simulink model "DBMPCC"  (R2022a)
settings: Solver=ode1  StartTime=0.0  StopTime=Inf  FixedStep=Ts  RelTol=1e-3  EnableMultiTasking=on
PostLoadFcn:
  | , if any(exist('dsrtsu_mdlpostloadfcn', 'file') ~= 0), dsrtsu_mdlpostloadfcn('Execute', bdroot); end,
InitFcn:
  | , if any(exist('rtifpga_mdlclblib', 'file') ~= 0), rtifpga_mdlclblib('Init', bdroot); end,
undefined symbols (not defined in the file): Ls, P, Ts
libraries: rtilib1104 x15, rtitasklib x1
settings Model: DSRTSU_INTERNAL_RTI_VER=600  DSRTSU_INTERNAL_RTI_TYPE=rti1104  DSRTSU_INTERNAL_RTIFPGA=180  DSRTSU_INTERNAL_RTISTBM_VER=1.4.4  SimulationMode=external  Creator=Admin  LastModifiedBy=acer
settings SolverCC: AlgebraicLoopSolver=TrustRegion
settings DataIOCC: LimitDataPoints=on  SaveFormat=Array  SignalLoggingSaveFormat=ModelDataLogs  ReturnWorkspaceOutputs=off
settings OptimizationCC: BlockReduction=off  OptimizeBlockIOStorage=off  BufferReuse=off  GlobalBufferReuse=off  ExpressionFolding=off  ExpressionDepthLimit=2147483647  LocalBlockOutputs=off  LifeSpan=inf
settings DebuggingCC: UnderspecifiedInitializationDetection=Classic  MergeDetectMultiDrivingBlocksExec=none  SolverPrmCheckMsg=warning  FcnCallInpInsideContextMsg=warning  UnconnectedInputMsg=warning  UnconnectedOutputMsg=warning  UnconnectedLineMsg=warning  StateNameClashWarn=warning  SFUnexpectedBacktrackingDiag=warning  SFNoUnconditionalDefaultTransitionDiag=warning  SFExecutionAtInitializationDiag=none  SFMachineParentedDataDiag=warning  ArithmeticOperatorsInVariantConditions=warning
settings HardwareCC: ProdBitPerPointer=32  ProdBitPerSizeT=32  ProdBitPerPtrDiffT=32  ProdLargestAtomicInteger=Integer  ProdEndianess=BigEndian  ProdWordSize=32  ProdHWDeviceType=Custom Processor->Custom  TargetIntDivRoundTo=Zero  TargetEndianess=BigEndian  TargetHWDeviceType=Custom Processor->Custom
settings ModelReferenceCC: PropagateSignalLabelsOutOfModel=off
settings SFSimCC: SimUseLocalCustomCode=off  MATLABDynamicMemAlloc=off  CustomCodeUndefinedFunction=UseInterfaceOnly
settings RTWCC: Description=dSPACE DS1104 Hardware Platform  SystemTargetFile=rti1104.tlc  MakeCommand=make_rti  TemplateMakefile=rti1104.tmf  RTWUseLocalCustomCode=off
settings CodeAppCC: StateflowObjectComments=on
settings STFCustomTargetCC: ParMdlRefBuildCompliant=on  GRTInterface=off  SystemTargetFile=rti1104.tlc
settings GRTTargetCC: TargetLangStandard=C89/C90 (ANSI)  CompOptLevelCompliant=off  ConcurrentExecutionCompliant=off  CombineOutputUpdateFcns=off  MatFileLogging=off  CPPClassGenCompliant=off  UseToolchainInfoCompliant=off  ExtModeMexFile=noextcomm
settings ConfigComp: CovMetricSettings=dw  CovSaveCumulativeToWorkspaceVar=on  CovSaveSingleToWorkspaceVar=on  CovExternalEMLEnable=off

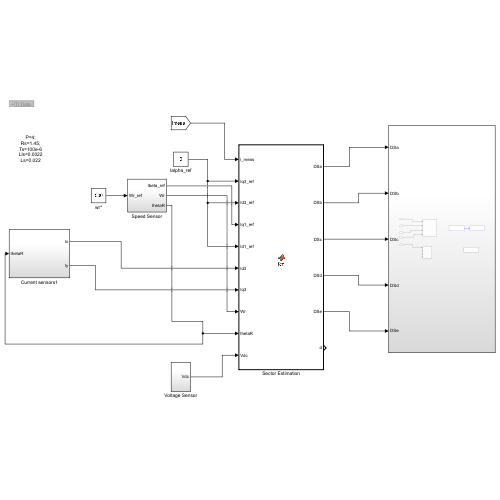
[thumbnail: Simulink's stored preview of the top-level diagram]
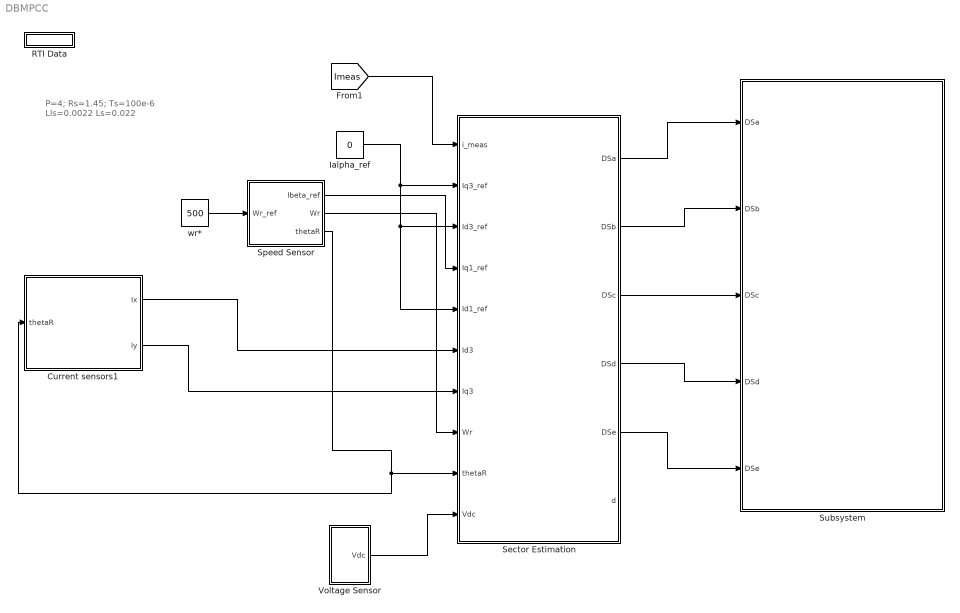
== system DBMPCC ==
  note: P=4;
      | Rs=1.45;
      | Ts=100e-6
      | Lls=0.0022
      | Ls=0.022
  Current sensors1 : Subsystem
  Ialpha_ref : Constant  Value=0
  RTI Data : Subsystem  Tag=struct('RTIDataServer',struct('RTIDataServerVs','2','RTIModelDescription','struct(''main'',''FP_CONV_PCC_SF_30V_PWM_n_duty_CurrErr'',''sub'','''',''isMp'',0)'))  LoadFcn="if exist('rtidc'), try,  rtidc('DataHostBlockClbLoad', gcbh); catch, disp(['Warning: ''LoadFcn'' for RTI Data block failed: ' lasterr]); end, end,"  mask(RTI_DATA_HOST){}
      mask help:
      | RTI Data Block.
      | This block is used by RTI to store internal model-dependent data.
      | Please keep this block on the root level of the model. Deleting this block will result in data loss.
      |
      | NEVER DELETE OR COPY THIS BLOCK!
      settings: CopyFcn="if exist('rtidc'), try,  rtidc('DataHostBlockClbCopy', gcbh); catch, disp(['Warning: ''CopyFcn'' for RTI Data block failed: ' lasterr]); end, end,"  DeleteFcn="if exist('rtidc'), try,  rtidc('DataHostBlockClbDelete', gcbh); catch, disp(['Warning: ''DeleteFcn'' for RTI Data block failed: ' lasterr]); end, end,"  ModelCloseFcn="if exist('rtidc'), try,  rtidc('DataHostBlockClbModelClose', gcbh); catch, disp(['Warning: ''ModelCloseFcn'' for RTI Data block failed: ' lasterr]); end, end,"  PreSaveFcn="if exist('rtidc'), try,  rtidc('DataHostBlockClbPreSave', gcbh); catch, disp(['Warning: ''PreSaveFcn'' for RTI Data block failed: ' lasterr]); end, end,"  PostSaveFcn="if exist('rtidc'), try,  rtidc('DataHostBlockClbPostSave', gcbh); catch, disp(['Warning: ''PostSaveFcn'' for RTI Data block failed: ' lasterr]); end, end,"  NameChangeFcn="if exist('rtidc'), try,  rtidc('DataHostBlockClbNameChange', gcbh); catch, disp(['Warning: ''NameChangeFcn'' for RTI Data block failed: ' lasterr]); end, end,"
      mask Help:
      | RTI Data Block.
      | This block is used by RTI to store internal model-dependent data.
      | Please keep this block on the root level of the model. Deleting this block will result in data loss.
      | 
      | NEVER DELETE OR COPY THIS BLOCK!
      mask Display:
      | text(0.5, 0.5, 'RTI Data', 'HorizontalAlignment', 'center');
      | plot([1 0]);
  Sector Estimation : MATLAB Function  TreatAsAtomicUnit=on  SystemSampleTime=Ts
  Speed Sensor : Subsystem
  Subsystem : Subsystem
  Voltage Sensor : Subsystem
  wr* : Constant  Value=500
  wires:
  Voltage Sensor/1(Vdc) -> Sector Estimation/10(Vdc)
  Ialpha_ref/1 -> Sector Estimation/2(Iq3_ref), Sector Estimation/3(Id3_ref), Sector Estimation/5(Id1_ref)
  wr*/1 -> Speed Sensor/1(Wr_ref)
  Speed Sensor/3(thetaR) -> Current sensors1/1(thetaR), Sector Estimation/9(thetaR)
  Speed Sensor/2(Wr) -> Sector Estimation/8(Wr)
  Speed Sensor/1(Ibeta_ref) -> Sector Estimation/4(Iq1_ref)
  [Imeas] -> Sector Estimation/1(i_meas)
  Current sensors1/1(Ix) -> Sector Estimation/6(Id3)
  Current sensors1/2(Iy) -> Sector Estimation/7(Iq3)
  Sector Estimation/1(DSa) -> Subsystem/1(DSa)
  Sector Estimation/2(DSb) -> Subsystem/2(DSb)
  Sector Estimation/3(DSc) -> Subsystem/3(DSc)
  Sector Estimation/4(DSd) -> Subsystem/4(DSd)
  Sector Estimation/5(DSe) -> Subsystem/5(DSe)

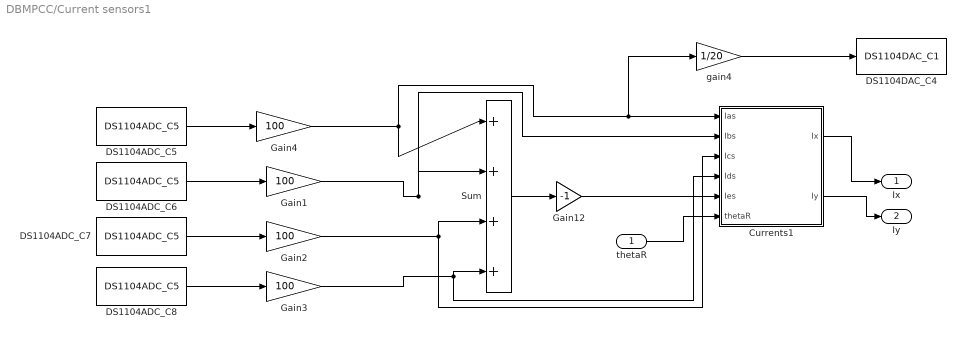
== system DBMPCC/Current sensors1 ==
  thetaR : Inport
  Currents1 : Subsystem
  DS1104ADC_C5 : rtilib1104/DS1104 MASTER PPC/DS1104ADC_C5  ChannelNo=5  TriggerMode=0  Reserved1=[]  Reserved2=[]  Reserved3=[]  Reserved4=[]  DialogFcn=gui1104adc  UnitName={ 'DS1104ADC_C' }  UnitValues={ 5 }  DSProperties=struct('RTI',struct('Version',uint32(1),'BlockType',struct('isSLSource',uint8(1),'isSLSink',uint8(0),'isHWSource',uint8(1),'isHWSink',uint8(0),'isSetup',uint8(0),'isInline',uint8(1),'isNonInline',uint8(0),'isInterrupt',uint8(0),'isChannelwise',uint8(1)),'IOBoardType','DS1104MASTER','UnitType','ADC','Identifier','ADC','DialogType','ML','BlockSet','NONE','SlaveProcessor','NONE'))
      settings: SourceProductName=dSPACE RTI1104
  DS1104ADC_C6 : rtilib1104/DS1104 MASTER PPC/DS1104ADC_C5  ChannelNo=6  TriggerMode=0  Reserved1=[]  Reserved2=[]  Reserved3=[]  Reserved4=[]  DialogFcn=gui1104adc  UnitName={ 'DS1104ADC_C' }  UnitValues={ 6 }  DSProperties=struct('RTI',struct('Version',uint32(1),'BlockType',struct('isSLSource',uint8(1),'isSLSink',uint8(0),'isHWSource',uint8(1),'isHWSink',uint8(0),'isSetup',uint8(0),'isInline',uint8(1),'isNonInline',uint8(0),'isInterrupt',uint8(0),'isChannelwise',uint8(1)),'IOBoardType','DS1104MASTER','UnitType','ADC','Identifier','ADC','DialogType','ML','BlockSet','NONE','SlaveProcessor','NONE'))
      settings: SourceProductName=dSPACE RTI1104
  DS1104ADC_C7 : rtilib1104/DS1104 MASTER PPC/DS1104ADC_C5  ChannelNo=7  TriggerMode=0  Reserved1=[]  Reserved2=[]  Reserved3=[]  Reserved4=[]  DialogFcn=gui1104adc  UnitName={ 'DS1104ADC_C' }  UnitValues={ 7 }  DSProperties=struct('RTI',struct('Version',uint32(1),'BlockType',struct('isSLSource',uint8(1),'isSLSink',uint8(0),'isHWSource',uint8(1),'isHWSink',uint8(0),'isSetup',uint8(0),'isInline',uint8(1),'isNonInline',uint8(0),'isInterrupt',uint8(0),'isChannelwise',uint8(1)),'IOBoardType','DS1104MASTER','UnitType','ADC','Identifier','ADC','DialogType','ML','BlockSet','NONE','SlaveProcessor','NONE'))
      settings: SourceProductName=dSPACE RTI1104
  DS1104ADC_C8 : rtilib1104/DS1104 MASTER PPC/DS1104ADC_C5  ChannelNo=8  TriggerMode=0  Reserved1=[]  Reserved2=[]  Reserved3=[]  Reserved4=[]  DialogFcn=gui1104adc  UnitName={ 'DS1104ADC_C' }  UnitValues={ 8 }  DSProperties=struct('RTI',struct('Version',uint32(1),'BlockType',struct('isSLSource',uint8(1),'isSLSink',uint8(0),'isHWSource',uint8(1),'isHWSink',uint8(0),'isSetup',uint8(0),'isInline',uint8(1),'isNonInline',uint8(0),'isInterrupt',uint8(0),'isChannelwise',uint8(1)),'IOBoardType','DS1104MASTER','UnitType','ADC','Identifier','ADC','DialogType','ML','BlockSet','NONE','SlaveProcessor','NONE'))
      settings: SourceProductName=dSPACE RTI1104
  DS1104DAC_C4 : rtilib1104/DS1104 MASTER PPC/DS1104DAC_C1  ChannelNo=4  InitValue=0  TermMode=0  TermValue=0  Reserved1=[]  Reserved2=[]  Reserved3=[]  Reserved4=[]  DialogFcn=gui1104dac  UnitName={ 'DS1104DAC_C'}  UnitValues={4}  DSProperties=struct('RTI',struct('Version',uint32(1),'BlockType',struct('isSLSource',uint8(0),'isSLSink',uint8(1),'isHWSource',uint8(0),'isHWSink',uint8(1),'isSetup',uint8(0),'isInline',uint8(1),'isNonInline',uint8(0),'isInterrupt',uint8(0),'isChannelwise',uint8(1)),'IOBoardType','DS1104MASTER','UnitType','DAC','Identifier','DAC','DialogType','ML','BlockSet','NONE','SlaveProcessor','NONE'))
      settings: SourceProductName=dSPACE RTI1104
  Gain{1..4} (4 alike) : Gain  Gain=100
  Gain12 : Gain  Gain=-1
  Sum : Sum  Inputs=|++++
  gain4 : Gain  Gain=1/20  SaturateOnIntegerOverflow=on  OutDataTypeStr=Inherit: Same as input  ParamDataTypeStr=Inherit: Same as input
  Ix : Outport
  Iy : Outport  Port=2
  wires:
  DS1104ADC_C5/1 -> Gain4/1
  DS1104ADC_C6/1 -> Gain1/1
  DS1104ADC_C7/1 -> Gain2/1
  DS1104ADC_C8/1 -> Gain3/1
  Sum/1 -> Gain12/1
  Gain12/1 -> Currents1/5(Ies)
  thetaR/1 -> Currents1/6(thetaR)
  Currents1/1(Ix) -> Ix/1
  Currents1/2(Iy) -> Iy/1
  Gain4/1 -> Sum/1, gain4/1, Currents1/1(Ias)
  Gain1/1 -> Currents1/2(Ibs), Sum/2
  Gain2/1 -> Currents1/3(Ics), Sum/3
  Gain3/1 -> Currents1/4(Ids), Sum/4
  gain4/1 -> DS1104DAC_C4/1

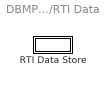
== system DBMPCC/RTI Data ==
  RTI Data Store : Subsystem  Tag="struct('private',struct('version',struct('dsVer',uint32(2),'dsVerCreation',uint32(2),'RTI',struct('ver','7.18','type','RTI1104')),'access',struct('type','Model','isPerm',1,'created',['03-Feb-2024 13:29:53'],'modified',['22-Jun-2024 12:50:59'],'location','')),'public',struct('main',struct('data',[]),'sub',struct('name',{{'FP_CONV_PCC_SF_30V_PWM_n_duty_CurrErr'}},'data',{{struct('TH',struct('thTaskInfo',struct('taskType',{'TIMER','HWINT','TMRINT','SWINT','GLINT'},'tasksNumOf',{1,0,0,0,0},'srcIds',{{'PWMINT'},{},{},{},{}},'taskNames',{{['Timer Task 1']},{},{},{},{}})),'th_tc',struct('dataType','TASK','taskGroupId','','taskGroupList',{{}},'taskSchedulingPolicy','FCFS','taskType','TIMER','blkh','FP_CONV_PCC_SF_30V_PWM_n_duty_CurrErr/Subsystem/DS1104SLAVE_PWMINT1','srcId','PWMINT','srcSgnName',['SLAVE-PWM-Interrupt with variable alignment'],'srcCpuName','','taskName',['Timer Task 1  [0.0001] s'],'taskNameDisplayExt','','smplTime',0.0001,'smplTimeOffs',0,'hasFixedPriority',0,'priority',1,'hasFixedOvc',0,'ovcType',1,'ovcMax',1),'tc_th',struct('dataType','TASK','taskGroupId','','taskGroupList',{{}},'taskSchedulingPolicy','FCFS','taskType','TIMER','blkh','FP_CONV_PCC_SF_30V_PWM_n_duty_CurrErr/Subsystem/DS1104SLAVE_PWMINT1','srcId','PWMINT','srcSgnName',['SLAVE-PWM-Interrupt with variable alignment'],'srcCpuName','','taskName',['Timer Task 1  [0.0001] s'],'taskNameDisplayExt','','smplTime',0.0001,'smplTimeOffs',0,'hasFixedPriority',0,'priority',1,'hasFixedOvc',0,'ovcType',1,'ovcMax',1))}})))"  mask(RTI_DATA_STORE){}
      mask help:
      | RTI Data Store Block. This block is used by RTI to store internal model dependent data. Deleting this block will result in data loss.
      |
      | NEVER DELETE, COPY, OR MODIFY THIS BLOCK!
      mask Help:
      | RTI Data Store Block. This block is used by RTI to store internal model dependent data. Deleting this block will result in data loss.
      | 
      | NEVER DELETE, COPY, OR MODIFY THIS BLOCK!
      mask Display: text(0.5, 0.5, ' ', 'HorizontalAlignment', 'center');

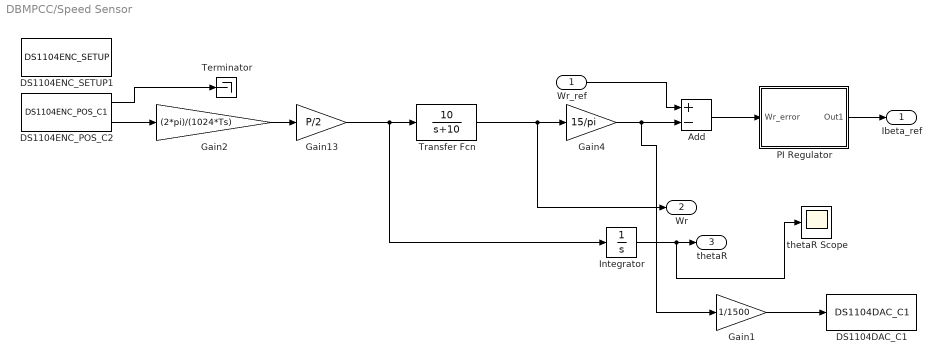
== system DBMPCC/Speed Sensor ==
  Wr_ref : Inport
  Add : Sum  Inputs=+-
  DS1104DAC_C1 : rtilib1104/DS1104 MASTER PPC/DS1104DAC_C1  ChannelNo=1  InitValue=0  TermMode=0  TermValue=0  Reserved1=[]  Reserved2=[]  Reserved3=[]  Reserved4=[]  DialogFcn=gui1104dac  UnitName={ 'DS1104DAC_C'}  UnitValues={ 1 }  DSProperties=struct('RTI',struct('Version',uint32(1),'BlockType',struct('isSLSource',uint8(0),'isSLSink',uint8(1),'isHWSource',uint8(0),'isHWSink',uint8(1),'isSetup',uint8(0),'isInline',uint8(1),'isNonInline',uint8(0),'isInterrupt',uint8(0),'isChannelwise',uint8(1)),'IOBoardType','DS1104MASTER','UnitType','DAC','Identifier','DAC','DialogType','ML','BlockSet','NONE','SlaveProcessor','NONE'))
      settings: SourceProductName=dSPACE RTI1104
  DS1104ENC_POS_C2 : rtilib1104/DS1104 MASTER PPC/DS1104ENC_POS_C1  ChannelNo=2  PosValue=0  Reserved1=[]  Reserved2=[]  Reserved3=[]  Reserved4=[]  DialogFcn=gui1104enc_pos  UnitName={'DS1104ENC_POS_C'}  UnitValues={ 2 }  DSProperties=struct('RTI',struct('Version',uint32(1),'BlockType',struct('isSLSource',uint8(1),'isSLSink',uint8(0),'isHWSource',uint8(1),'isHWSink',uint8(0),'isSetup',uint8(0),'isInline',uint8(1),'isNonInline',uint8(0),'isInterrupt',uint8(0),'isChannelwise',uint8(1)),'IOBoardType','DS1104MASTER','UnitType','ENC','Identifier','ENCPOSCH','DialogType','ML','BlockSet','NONE','SlaveProcessor','NONE'))
      settings: SourceProductName=dSPACE RTI1104
  DS1104ENC_SETUP1 : rtilib1104/DS1104 MASTER PPC/DS1104ENC_SETUP  Reserved1=[]  Reserved2=[]  Reserved3=[]  Reserved4=[]  DialogFcn=gui1104enc_setup  UnitName={'DS1104ENC_SETUP'}  UnitValues={ [] }  DSProperties=struct('RTI',struct('Version',uint32(1),'BlockType',struct('isSLSource',uint8(0),'isSLSink',uint8(0),'isHWSource',uint8(0),'isHWSink',uint8(0),'isSetup',uint8(0),'isInline',uint8(1),'isNonInline',uint8(0),'isInterrupt',uint8(0),'isChannelwise',uint8(0)),'IOBoardType','DS1104MASTER','UnitType','ENC','Identifier','ENCSETUP','DialogType','ML','BlockSet','NONE','SlaveProcessor','NONE'))
      settings: SourceProductName=dSPACE RTI1104  SignalType=[0 0]
  Gain1 : Gain  Gain=1/1500
  Gain13 : Gain  Gain=P/2
  Gain2 : Gain  Gain=(2*pi)/(1024*Ts)
  Gain4 : Gain  Gain=15/pi
  Integrator : Integrator
  PI Regulator : Subsystem
  Terminator : Terminator
  Transfer Fcn : TransferFcn  Numerator=[10]  Denominator=[1 10]
  thetaR Scope : Scope
  Ibeta_ref : Outport
  Wr : Outport  Port=2
  thetaR : Outport  Port=3
  wires:
  DS1104ENC_POS_C2/2 -> Gain2/1
  Gain2/1 -> Gain13/1
  DS1104ENC_POS_C2/1 -> Terminator/1
  Wr_ref/1 -> Add/1
  Add/1 -> PI Regulator/1(Wr_error)
  PI Regulator/1(Out1) -> Ibeta_ref/1
  Integrator/1 -> thetaR Scope/1, thetaR/1
  Gain13/1 -> Transfer Fcn/1, Integrator/1
  Transfer Fcn/1 -> Wr/1, Gain4/1
  Gain1/1 -> DS1104DAC_C1/1
  Gain4/1 -> Gain1/1, Add/2

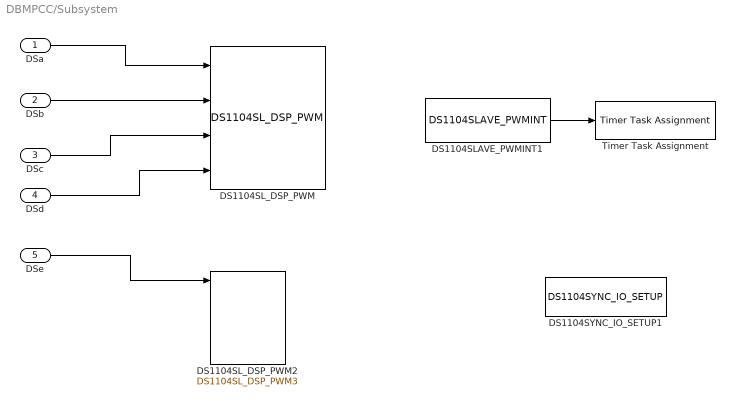
== system DBMPCC/Subsystem ==
  DSa : Inport
  DSb : Inport  Port=2
  DSc : Inport  Port=3
  DSd : Inport  Port=4
  DSe : Inport  Port=5
  DS1104SLAVE_PWMINT1 : rtilib1104/DS1104 SLAVE DSP/DS1104SLAVE_PWMINT  Parameters=[]  TDef=[]  BoardIntNo=[]  InterruptName=[]  Delay=[]  DialogFcn=[]  Reserved1=[]  Reserved2=[]  Reserved3=[]  Reserved4=[]  Revision=[]  UnitName=[]  UnitValues=[]  DSProperties=struct('RTI',struct('Version',uint32(530),'IOBoardType','DS1104SLAVE','SlaveProcessor','F240','UnitType','HWINT','Identifier','PWMINT','BlockType',struct('isSLSource',uint8(1),'isSLSink',uint8(0),'isHWSource',uint8(1),'isHWSink',uint8(0),'isSetup',uint8(0),'isInline',uint8(1),'isNonInline',uint8(0),'isInterrupt',uint8(1),'isChannelwise',uint8(0)),'DialogType','ML','BlockSet','NONE','RelationId',struct('TH',struct('BlockId','HWINT'))))  RTIBlockInterface=struct('BlockName',struct('Token',{{'DS1104SLAVE_PWMINT'}}),'BlockDisplay',{{['DS1104SLAVE Board \nPWM-Interrupt'],'center'}},'DialogFcn','rti110xhwintgui','OutputPortsActive',1,'OutputPortsWidth',int32(1),'FunctionCall',uint32(0),'OutputPortsName',{{[' ']}},'IconTransparency','on','InitLevel',3,'Options',{{'SS_OPTION_FORCE_NONINLINED_FCNCALL','SS_OPTION_ASYNCHRONOUS_INTERRUPT'}},'OutputPortsDataType',{{'SS_FCN_CALL'}})  RTIBlockParameters=struct('ThIntNo',{{10,'OFF',[]}},'IntDelay',{{0.01,'ON',[1e-6 1]}},'ThSrcSgnName',{{['SLAVE-PWM-Interrupt with variable alignment'],'OFF',[]}},'TLCFileName',{{'rti1104slave_pwm_interrupt','OFF',[]}},'ThBlk',{{['struct(''blkh'',''FP_CONV_PCC_SF_30V_PWM_n_duty_CurrErr/Subsystem/DS1104SLAVE_PWMINT1'',''srcId'',''PWMINT'',''srcSgnId'',''PWMINT'',''intervalTmrBlockId'',[],''srcSgnName'',[''SLAVE-PWM-Interrupt with variable alignment''],''srcCpuId'','''',''isSrcCpu'',1,''isTargetCpu'',1,''srcOnMasterCpu'',1,''boardType'','''',''boardTypeNo'','''',''boardNo'',1,''intNo'',0,''subIntNo'',-1,''period'',0,''entryPoint'',''rti_PWMINT'',''blockName'',''DS1104SLAVE_PWMINT1'',''taskNameDisplayExt'','''',''taskType'',''HWINT'',''groupId'',''PWMINT'',''hookFcn'',''NULL'',''isTimerTaskSrc'',1,''service'','''',''mpBlkId'','''',''taskPriorityPreConfig'',''none'',''taskPriority'',-1,''taskSortWeighting'',[],''taskSchedulingPolicy'',''FCFS'',''taskOvrPreConfig'',''none'',''taskOvrStrategy'',1,''taskOvrQueueSize'',1,''taskVisibility'',''on'',''taskGroupId'','''',''taskGroupDisplayOrder'',[],''serviceDynamicGen'',0,''disableCodeGen'',0,''boardBase'',''0'',''noBoardBase'','''')'],'OFF',[]}},'PHSBoardBaseId',{{'DSXXXX','OFF',[]}})  RTISFcnParameters=struct('IntDelay','double','ThBlk','struct','ThIntNo','int32','TLCFileName','char','PHSBoardBaseId','char')  RTIBlockParaDefault=struct('ThIntNo',10,'IntDelay',2^-1,'ThSrcSgnName',['SLAVE-PWM-Interrupt with none delay'],'TLCFileName','rti1104slave_pwm_interrupt','ThBlk',['struct(''srcSgnId'', '''')'],'PHSBoardBaseId','DSXXXX')
      settings: SourceProductName=dSPACE RTI1104
  DS1104SL_DSP_PWM : rtilib1104/DS1104 SLAVE DSP/DS1104SL_DSP_PWM  Parameters=[]  TDef=[]  BoardType=[]  PwmMode=[]  Frequency=[]  InitValue=[]  TermMode=[]  TermValue=[]  Polarity=[]  DialogFcn=[]  Reserved1=[]  Reserved2=[]  Reserved3=[]  Reserved4=[]  Revision=[]  UnitName=[]  UnitValues=[]  DSProperties=struct('RTI',struct('Version',uint32(2),'BlockType',struct('isSLSource',uint8(0),'isSLSink',uint8(1),'isHWSource',uint8(0),'isHWSink',uint8(1),'isSetup',uint8(0),'isInline',uint8(1),'isNonInline',uint8(0),'isInterrupt',uint8(0),'isChannelwise',uint8(0)),'IOBoardType','DS1104SLAVE','UnitType','PWM','Identifier','PWM','DialogType','ML','BlockSet','NONE','SlaveProcessor','F240'))  RTIBlockInterface=struct('InputPortsActive',[1 1 1 1],'InputPortsWidth',int32([1 1 1 1]),'InputPortsName',{{['PWM Channel 1'],['PWM Channel 2'],['PWM Channel 3'],['PWM Channel 4']}},'IWork',{{{'',uint32(4)}}},'DialogFcn','rti1104slavepwmgui','InitLevel',1,'BlockDisplay',{{'','auto'}},'IconTransparency','on','MultiSFcn',4,'BlockName',struct('Token',{{'DS1104SL_DSP_PWM'}}))  RTIBlockParameters=struct('PWMSymmetryMode',{{2,'OFF',[]}},'PWMFrequency',{{'1/Ts','OFF',[]}},'PWMPolarityMode',{{[1 1 1 1 1],'OFF',[]}},'ChannelNo',{{[1 2 3 4],'OFF',[]}},'SuspendModeInit',{{[1 1 1 1 1],'OFF',[]}},'TTLModeInit',{{[2 2 2 2 2],'OFF',[]}},'DutyCycleInitValueCh1',{{'0.5','OFF',[]}},'DutyCycleInitValueCh2',{{'0.5','OFF',[]}},'DutyCycleInitValueCh3',{{'0.5','OFF',[]}},'DutyCycleInitValueCh4',{{'0.5','OFF',[]}},'DutyCycleInitValueCh5',{{'0.5','OFF',[]}},'EnablePWMStop',{{[0 0 0 0 0],'OFF',[]}},'SuspendModeTerm',{{[0 1 1 1 1],'OFF',[]}},'TTLModeTerm',{{[2 2 2 2 2],'OFF',[]}},'DutyCycleTermValueCh1',{{'0.5','OFF',[]}},'DutyCycleTermValueCh2',{{'0.5','OFF',[]}},'DutyCycleTermValueCh3',{{'0.5','OFF',[]}},'DutyCycleTermValueCh4',{{'0.5','OFF',[]}},'DutyCycleTermValueCh5',{{'0.5','OFF',[]}},'TLCFileName',{{'rti1104pwm','OFF',[]}})  RTISFcnParameters=struct('PWMSymmetryMode','double','PWMFrequency','double','PWMPolarityMode','double','ChannelNo','double','SuspendModeInit','double','TTLModeInit','double','DutyCycleInitValueCh1','double','DutyCycleInitValueCh2','double','DutyCycleInitValueCh3','double','DutyCycleInitValueCh4','double','EnablePWMStop','double','SuspendModeTerm','double','TTLModeTerm','double','DutyCycleTermValueCh1','double','DutyCycleTermValueCh2','double','DutyCycleTermValueCh3','double','DutyCycleTermValueCh4','double','TLCFileName','char')  RTIBlockParaDefault=struct('PWMSymmetryMode',1,'PWMFrequency',100,'PWMPolarityMode',[1 1 1 1 1],'ChannelNo',[1 2 3 4],'SuspendModeInit',[1 1 1 1 1],'TTLModeInit',[2 2 2 2 2],'DutyCycleInitValueCh1',2^-1,'DutyCycleInitValueCh2',2^-1,'DutyCycleInitValueCh3',2^-1,'DutyCycleInitValueCh4',2^-1,'DutyCycleInitValueCh5',2^-1,'EnablePWMStop',[1 1 1 1 0],'SuspendModeTerm',[1 1 1 1 1],'TTLModeTerm',[2 2 2 2 2],'DutyCycleTermValueCh1',2^-1,'DutyCycleTermValueCh2',2^-1,'DutyCycleTermValueCh3',2^-1,'DutyCycleTermValueCh4',2^-1,'DutyCycleTermValueCh5',2^-1,'TLCFileName','rti1104pwm')
      settings: SourceProductName=dSPACE RTI1104
  DS1104SL_DSP_PWM2 : rtilib1104/DS1104 SLAVE DSP/DS1104SL_DSP_PWM3  Parameters=[]  TDef=[]  BoardType=[]  PwmMode=[]  Frequency=[]  DeadBand=[]  InitValue=[]  TermMode=[]  TermValue=[]  IntDelay=[]  DialogFcn=[]  Reserved1=[]  Reserved2=[]  Reserved3=[]  Reserved4=[]  Revision=[]  UnitName=[]  UnitValues=[]  DSProperties=struct('RTI',struct('Version',uint32(2),'BlockType',struct('isSLSource',uint8(0),'isSLSink',uint8(1),'isHWSource',uint8(0),'isHWSink',uint8(1),'isSetup',uint8(0),'isInline',uint8(1),'isNonInline',uint8(0),'isInterrupt',uint8(0),'isChannelwise',uint8(0)),'IOBoardType','DS1104SLAVE','UnitType','PWM','Identifier','PWM3','DialogType','ML','BlockSet','NONE','SlaveProcessor','F240'))  RTIBlockInterface=struct('InputPortsActive',[1 1 1 1],'InputPortsWidth',int32([1 1 1 1]),'InputPortsName',{{['Duty cycle a'],['Duty cycle b'],['Duty cycle c'],['PWM Stop']}},'IWork',{{{'',uint32(1)}}},'DialogFcn','rti1104slavepwm3gui','InitLevel',1,'BlockDisplay',{{'','auto'}},'IconTransparency','on','BlockName',struct('Token',{{'DS1104SL_DSP_PWM3'}}))  RTIBlockParameters=struct('PWMFrequency',{{'1/Ts','OFF',[]}},'PWMDeadband',{{'0','OFF',[]}},'PWMPolarityMode',{{[1 1 1 1],'OFF',[]}},'PWMPolarityInvMode',{{[2 2 2 2],'OFF',[]}},'SuspendModeInit',{{[1 1 1],'OFF',[]}},'TTLModeInit',{{[2 2 2],'OFF',[]}},'TTLModeInitNOT',{{[1 1 1],'OFF',[]}},'DutyCycleInitValueCh1',{{'0.5','OFF',[]}},'DutyCycleInitValueCh2',{{'0.5','OFF',[]}},'DutyCycleInitValueCh3',{{'0.5','OFF',[]}},'EnablePWMStop',{{1,'OFF',[]}},'SuspendModeTerm',{{[1 1 1],'OFF',[]}},'TTLModeTerm',{{[2 2 2],'OFF',[]}},'TTLModeTermNOT',{{[1 1 1],'OFF',[]}},'DutyCycleTermValueCh1',{{'0.5','OFF',[]}},'DutyCycleTermValueCh2',{{'0.5','OFF',[]}},'DutyCycleTermValueCh3',{{'0.5','OFF',[]}},'TLCFileName',{{'rti1104pwm3','OFF',[]}})  RTISFcnParameters=struct('PWMFrequency','double','PWMDeadband','double','PWMPolarityMode','double','PWMPolarityInvMode','double','SuspendModeInit','double','TTLModeInit','double','TTLModeInitNOT','double','DutyCycleInitValueCh1','double','DutyCycleInitValueCh2','double','DutyCycleInitValueCh3','double','EnablePWMStop','double','SuspendModeTerm','double','TTLModeTerm','double','TTLModeTermNOT','double','DutyCycleTermValueCh1','double','DutyCycleTermValueCh2','double','DutyCycleTermValueCh3','double','TLCFileName','char')  RTIBlockParaDefault=struct('PWMFrequency',100,'PWMDeadband',50,'PWMPolarityMode',[1 1 1 1],'PWMPolarityInvMode',[2 2 2 2],'SuspendModeInit',[1 1 1],'TTLModeInit',[2 2 2],'TTLModeInitNOT',[1 1 1],'DutyCycleInitValueCh1',2^-1,'DutyCycleInitValueCh2',2^-1,'DutyCycleInitValueCh3',2^-1,'EnablePWMStop',1,'SuspendModeTerm',[1 1 1],'TTLModeTerm',[2 2 2],'TTLModeTermNOT',[1 1 1],'DutyCycleTermValueCh1',2^-1,'DutyCycleTermValueCh2',2^-1,'DutyCycleTermValueCh3',2^-1,'TLCFileName','rti1104pwm3')
      settings: SourceProductName=dSPACE RTI1104
  DS1104SYNC_IO_SETUP1 : rtilib1104/DS1104 MASTER PPC/DS1104SYNC_IO_SETUP  DSProperties=struct('RTI',struct('Version',uint32(1),'BlockType',struct('isSLSource',uint8(0),'isSLSink',uint8(0),'isHWSource',uint8(0),'isHWSink',uint8(0),'isSetup',uint8(1),'isInline',uint8(1),'isNonInline',uint8(0),'isInterrupt',uint8(0),'isChannelwise',uint8(0)),'IOBoardType','DS1104MASTER','UnitType','SETUP','Identifier','SYNCSETUP','DialogType','ML','BlockSet','NONE','SlaveProcessor','NONE'))  RTIBlockInterface=struct('OutputPortsActive',0,'OutputPortsWidth',int32(0),'DialogFcn','gui1104mastersyncsetup','InitLevel',1,'BlockDisplay',{{['Master Sync IO Setup'],'center'}},'IconTransparency','off','BlockName',struct('Token',{{'DS1104SYNC_IO_SETUP'}}))  RTIBlockParameters=struct('TriggerSource',{{1,'OFF',[]}},'SyncIn',{{2,'OFF',[]}},'SyncOut',{{2,'OFF',[]}},'SyncADC',{{[0 0 0 0 0],'OFF',[]}},'SyncDAC',{{0,'OFF',[]}},'SyncInc',{{[0 0],'OFF',[]}},'TLCFileName',{{'rti1104mastersyncsetup','OFF',[]}})  RTISFcnParameters=struct('TriggerSource','int32','SyncIn','int32','SyncOut','int32','SyncADC','int32','SyncDAC','int32','SyncInc','int32','TLCFileName','char')  RTIBlockParaDefault=struct('TriggerSource',1,'SyncIn',1,'SyncOut',1,'SyncADC',[0 0 0 0 0],'SyncDAC',0,'SyncInc',[0 0],'TLCFileName','rti1104mastersyncsetup')
      settings: SourceProductName=dSPACE RTI1104
  Timer Task Assignment : rtitasklib/Timer Task Assignment  Reserved2=[]  Reserved3=[]  Reserved4=[]  DSProperties=struct('RTI',struct('Version',uint32(2),'BlockType',struct('isSLSource',uint8(0),'isSLSink',uint8(1),'isHWSource',uint8(0),'isHWSink',uint8(0),'isSetup',uint8(0),'isInline',uint8(1),'isNonInline',uint8(0),'isInterrupt',uint8(0),'isChannelwise',uint8(0)),'IOBoardType','INTLIB','UnitType','TTASSIGN','Identifier','TTASSIGN','DialogType','SL','BlockSet','NONE','SlaveProcessor','NONE','RelationId',struct('TH',struct('BlockId','TTASSIGN'))))
  wires:
  DSc/1 -> DS1104SL_DSP_PWM/3
  DSe/1 -> DS1104SL_DSP_PWM2/1
  DSa/1 -> DS1104SL_DSP_PWM/1
  DSb/1 -> DS1104SL_DSP_PWM/2
  DSd/1 -> DS1104SL_DSP_PWM/4
  DS1104SLAVE_PWMINT1/1 -> Timer Task Assignment/1

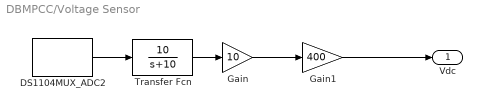
== system DBMPCC/Voltage Sensor ==
  DS1104MUX_ADC2 : rtilib1104/DS1104 MASTER PPC/DS1104MUX_ADC  ChannelNos=1  TriggerMode=0  Reserved1=[]  Reserved2=[]  Reserved3=[]  Reserved4=[]  DialogFcn=gui1104mux_adc  UnitName={ 'DS1104MUX_ADC' }  UnitValues={ [] }  DSProperties=struct('RTI',struct('Version',uint32(1),'BlockType',struct('isSLSource',uint8(1),'isSLSink',uint8(0),'isHWSource',uint8(1),'isHWSink',uint8(0),'isSetup',uint8(0),'isInline',uint8(1),'isNonInline',uint8(0),'isInterrupt',uint8(0),'isChannelwise',uint8(0)),'IOBoardType','DS1104MASTER','UnitType','ADC','Identifier','ADCMUX','DialogType','ML','BlockSet','NONE','SlaveProcessor','NONE'))
      settings: SourceProductName=dSPACE RTI1104
  Gain : Gain  Gain=10
  Gain1 : Gain  Gain=400
  Transfer Fcn : TransferFcn  Numerator=[10]  Denominator=[1 10]
  Vdc : Outport
  wires:
  Gain/1 -> Gain1/1
  Transfer Fcn/1 -> Gain/1
  Gain1/1 -> Vdc/1
  DS1104MUX_ADC2/1 -> Transfer Fcn/1

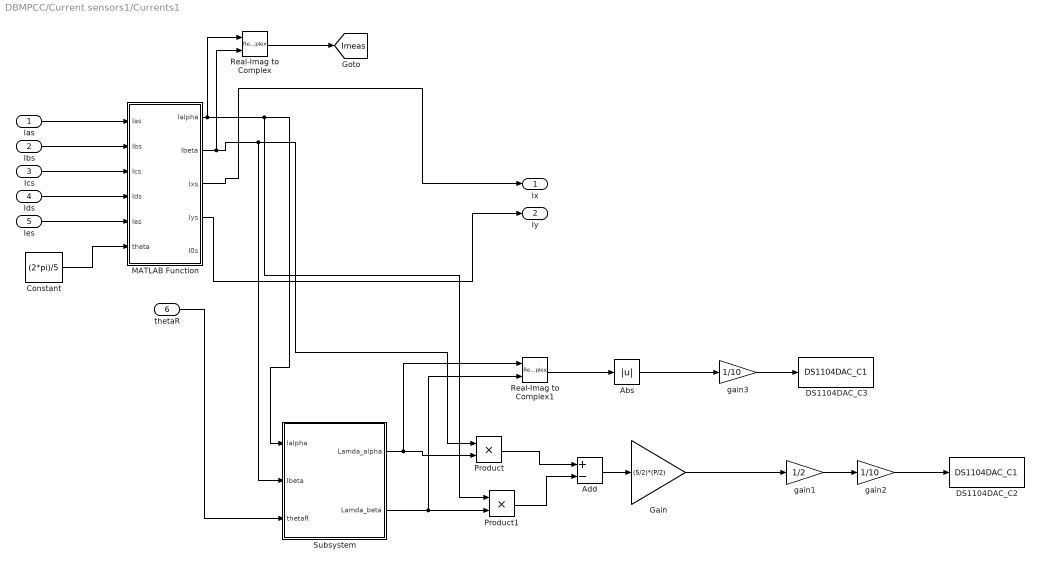
== system DBMPCC/Current sensors1/Currents1 ==
  Ias : Inport
  Ibs : Inport  Port=2
  Ics : Inport  Port=3
  Ids : Inport  Port=4
  Ies : Inport  Port=5
  thetaR : Inport  Port=6
  Abs : Abs  SaturateOnIntegerOverflow=off
  Add : Sum  Inputs=+-
  Constant : Constant  Value=(2*pi)/5
  DS1104DAC_C2 : rtilib1104/DS1104 MASTER PPC/DS1104DAC_C1  ChannelNo=2  InitValue=0  TermMode=0  TermValue=0  Reserved1=[]  Reserved2=[]  Reserved3=[]  Reserved4=[]  DialogFcn=gui1104dac  UnitName={ 'DS1104DAC_C'}  UnitValues={ 2 }  DSProperties=struct('RTI',struct('Version',uint32(1),'BlockType',struct('isSLSource',uint8(0),'isSLSink',uint8(1),'isHWSource',uint8(0),'isHWSink',uint8(1),'isSetup',uint8(0),'isInline',uint8(1),'isNonInline',uint8(0),'isInterrupt',uint8(0),'isChannelwise',uint8(1)),'IOBoardType','DS1104MASTER','UnitType','DAC','Identifier','DAC','DialogType','ML','BlockSet','NONE','SlaveProcessor','NONE'))
      settings: SourceProductName=dSPACE RTI1104
  DS1104DAC_C3 : rtilib1104/DS1104 MASTER PPC/DS1104DAC_C1  ChannelNo=3  InitValue=0  TermMode=0  TermValue=0  Reserved1=[]  Reserved2=[]  Reserved3=[]  Reserved4=[]  DialogFcn=gui1104dac  UnitName={ 'DS1104DAC_C'}  UnitValues={ 3 }  DSProperties=struct('RTI',struct('Version',uint32(1),'BlockType',struct('isSLSource',uint8(0),'isSLSink',uint8(1),'isHWSource',uint8(0),'isHWSink',uint8(1),'isSetup',uint8(0),'isInline',uint8(1),'isNonInline',uint8(0),'isInterrupt',uint8(0),'isChannelwise',uint8(1)),'IOBoardType','DS1104MASTER','UnitType','DAC','Identifier','DAC','DialogType','ML','BlockSet','NONE','SlaveProcessor','NONE'))
      settings: SourceProductName=dSPACE RTI1104
  Gain : Gain  Gain=(5/2)*(P/2)
  MATLAB Function : MATLAB Function  TreatAsAtomicUnit=on
  Product : Product
  Product1 : Product
  Real-Imag to Complex : RealImagToComplex
  Real-Imag to Complex1 : RealImagToComplex
  Subsystem : Subsystem
  gain1 : Gain  Gain=1/2  SaturateOnIntegerOverflow=on  OutDataTypeStr=Inherit: Same as input  ParamDataTypeStr=Inherit: Same as input
  gain2 : Gain  Gain=1/10  SaturateOnIntegerOverflow=on  OutDataTypeStr=Inherit: Same as input  ParamDataTypeStr=Inherit: Same as input
  gain3 : Gain  Gain=1/10  SaturateOnIntegerOverflow=on  OutDataTypeStr=Inherit: Same as input  ParamDataTypeStr=Inherit: Same as input
  Ix : Outport
  Iy : Outport  Port=2
  tag scope: Imeas=global
  wires:
  Constant/1 -> MATLAB Function/6(theta)
  MATLAB Function/1(Ialpha) -> Real-Imag to Complex/1, Product1/1, Subsystem/1(Ialpha)
  MATLAB Function/2(Ibeta) -> Real-Imag to Complex/2, Product/1, Subsystem/2(Ibeta)
  MATLAB Function/3(Ixs) -> Ix/1
  MATLAB Function/4(Iys) -> Iy/1
  Ibs/1 -> MATLAB Function/2(Ibs)
  Ics/1 -> MATLAB Function/3(Ics)
  Ids/1 -> MATLAB Function/4(Ids)
  Ies/1 -> MATLAB Function/5(Ies)
  Real-Imag to Complex/1 -> [Imeas]
  thetaR/1 -> Subsystem/3(thetaR)
  Subsystem/2(Lamda_beta) -> Real-Imag to Complex1/2, Product1/2
  Product/1 -> Add/1
  Product1/1 -> Add/2
  Add/1 -> Gain/1
  gain1/1 -> gain2/1
  gain2/1 -> DS1104DAC_C2/1
  Gain/1 -> gain1/1
  Real-Imag to Complex1/1 -> Abs/1
  Abs/1 -> gain3/1
  gain3/1 -> DS1104DAC_C3/1
  Ias/1 -> MATLAB Function/1(Ias)
  Subsystem/1(Lamda_alpha) -> Real-Imag to Complex1/1, Product/2

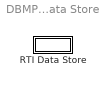
== system DBMPCC/RTI Data/RTI Data Store ==
  RTI Data Store : Subsystem  mask(RTI_DATA_STORE){}
      mask help:
      | RTI Data Store Block. This block is used by RTI to store internal model dependent data. Deleting this block will result in data loss.
      |
      | NEVER DELETE, COPY, OR MODIFY THIS BLOCK!
      mask Help:
      | RTI Data Store Block. This block is used by RTI to store internal model dependent data. Deleting this block will result in data loss.
      | 
      | NEVER DELETE, COPY, OR MODIFY THIS BLOCK!
      mask Display: text(0.5, 0.5, ' ', 'HorizontalAlignment', 'center');

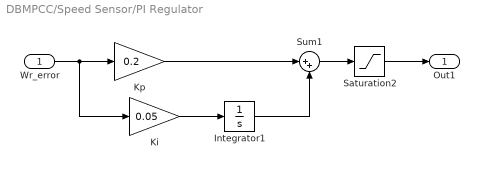
== system DBMPCC/Speed Sensor/PI Regulator ==
  Wr_error : Inport
  Integrator1 : Integrator  LimitOutput=on  UpperSaturationLimit=10  LowerSaturationLimit=-10
  Ki : Gain  Gain=0.05
  Kp : Gain  Gain=0.2
  Saturation2 : Saturate  UpperLimit=10  LowerLimit=-10
  Sum1 : Sum  Inputs=|++
  Out1 : Outport
  wires:
  Ki/1 -> Integrator1/1
  Kp/1 -> Sum1/1
  Integrator1/1 -> Sum1/2
  Sum1/1 -> Saturation2/1
  Wr_error/1 -> Kp/1, Ki/1
  Saturation2/1 -> Out1/1

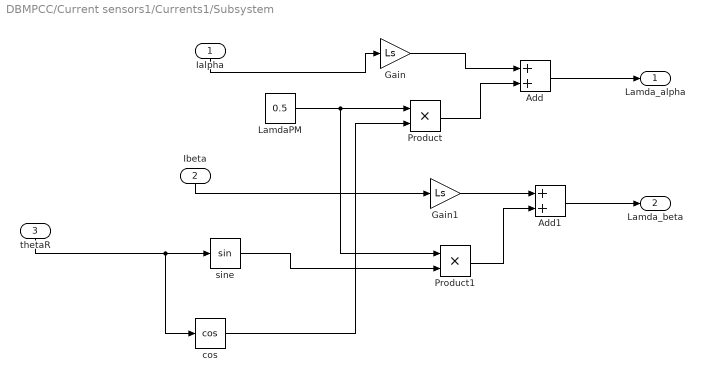
== system DBMPCC/Current sensors1/Currents1/Subsystem ==
  Ialpha : Inport
  Ibeta : Inport  Port=2
  thetaR : Inport  Port=3
  Add : Sum
  Add1 : Sum
  Gain : Gain  Gain=Ls
  Gain1 : Gain  Gain=Ls
  LamdaPM : Constant  Value=0.5
  Product : Product
  Product1 : Product
  cos : Trigonometry  Operator=cos
  sine : Trigonometry
  Lamda_alpha : Outport
  Lamda_beta : Outport  Port=2
  wires:
  Gain1/1 -> Add1/1
  Ialpha/1 -> Gain/1
  Ibeta/1 -> Gain1/1
  thetaR/1 -> sine/1, cos/1
  Gain/1 -> Add/1
  Add1/1 -> Lamda_beta/1
  Add/1 -> Lamda_alpha/1
  LamdaPM/1 -> Product1/1, Product/1
  Product1/1 -> Add1/2
  Product/1 -> Add/2
  sine/1 -> Product1/2
  cos/1 -> Product/2

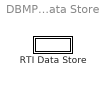
== system DBMPCC/RTI Data/RTI Data Store/RTI Data Store ==
  RTI Data Store : Subsystem  mask(RTI_DATA_STORE){}
      mask help:
      | RTI Data Store Block. This block is used by RTI to store internal model dependent data. Deleting this block will result in data loss.
      |
      | NEVER DELETE, COPY, OR MODIFY THIS BLOCK!
      mask Help:
      | RTI Data Store Block. This block is used by RTI to store internal model dependent data. Deleting this block will result in data loss.
      | 
      | NEVER DELETE, COPY, OR MODIFY THIS BLOCK!
      mask Display: text(0.5, 0.5, ' ', 'HorizontalAlignment', 'center');

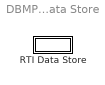
== system DBMPCC/RTI Data/RTI Data Store/RTI Data Store/RTI Data Store ==
  RTI Data Store : Subsystem  mask(RTI_DATA_STORE){}
      mask help:
      | RTI Data Store Block. This block is used by RTI to store internal model dependent data. Deleting this block will result in data loss.
      |
      | NEVER DELETE, COPY, OR MODIFY THIS BLOCK!
      mask Help:
      | RTI Data Store Block. This block is used by RTI to store internal model dependent data. Deleting this block will result in data loss.
      | 
      | NEVER DELETE, COPY, OR MODIFY THIS BLOCK!
      mask Display: text(0.5, 0.5, ' ', 'HorizontalAlignment', 'center');

== system DBMPCC/RTI Data/RTI Data Store/RTI Data Store/RTI Data Store/RTI Data Store ==

== matlab function DBMPCC/Current sensors1/Currents1/MATLAB Function ==
  data: Ias input; Ialpha output; Ibs input; Ics input; Ids input; Ies input; theta input; Ibeta output; Ixs output; Iys output; I0s output
function [Ialpha,Ibeta,Ixs,Iys,I0s] = fcn(Ias,Ibs,Ics,Ids,Ies,theta)
Ialpha=(2/5)*(Ias*cos(0)+Ibs*cos(theta)+Ics*cos(2*theta)+Ids*cos(3*theta)+Ies*cos(4*theta));
Ibeta=(2/5)*(Ias*sin(0)+Ibs*sin(theta)+Ics*sin(2*theta)+Ids*sin(3*theta)+Ies*sin(4*theta));
Ixs=(2/5)*(Ias*cos(0)+Ibs*cos(3*theta)+Ics*cos(6*theta)+Ids*cos(9*theta)+Ies*cos(12*theta));
Iys=(2/5)*(Ias*sin(0)+Ibs*sin(3*theta)+Ics*sin(6*theta)+Ids*sin(9*theta)+Ies*sin(12*theta));
I0s=(2/5)*(1/2)*(Ias+Ibs+Ics+Ids+Ies);

== matlab function DBMPCC/Sector Estimation ==
  data: i_meas input; Iq3_ref input; Id3_ref input; Iq1_ref input; DSa output; DSb output; Id1_ref input; Id3 input; Iq3 input; Wr input; thetaR input; Vdc input; DSc output; DSd output; DSe output; d output
 function [DSa,DSb,DSc,DSd,DSe,d] = fcn(i_meas,Iq3_ref,Id3_ref,Iq1_ref,Id1_ref,Id3,Iq3,Wr,thetaR,Vdc)
Ts =100e-6;
Rs=1.45;
Ls=0.022;
Lls=0.0022;
Lamda_PM=0.5;
V1=2/5*Vdc*(1.6180+1j*0);
V2=2/5*Vdc*(1.3090+1j*0.9510);
V3=2/5*Vdc*(0.5+1j*1.5388);
V4=2/5*Vdc*(-0.5+1j*1.5388);
V5=2/5*Vdc*(-1.3090+1j*0.9510);
V6=2/5*Vdc*(-1.6180+1j*0);
V7=2/5*Vdc*(-1.3090-1j*0.9510);
V8=2/5*Vdc*(-0.5-1j*1.5388);
V9=2/5*Vdc*(0.5-1j*1.5388);
V10=2/5*Vdc*(1.3090-1j*0.9510);
V11=2/5*Vdc*(1+1j*0);
V12=2/5*Vdc*(0.8090+1j*0.5877);
V13=2/5*Vdc*(0.3090+1j*0.9510);
V14=2/5*Vdc*(-0.3090+1j*0.9510);
V15=2/5*Vdc*(-0.8090+1j*0.5877);
V16=2/5*Vdc*(-1+1j*0);
V17=2/5*Vdc*(-0.8090-1j*0.5877);
V18=2/5*Vdc*(-0.3090-1j*0.9510);
V19=2/5*Vdc*(0.3090-1j*0.9510);
V20=2/5*Vdc*(0.8090-1j*0.5877);
V21=2/5*Vdc*(0.6180+1j*0);
V22=2/5*Vdc*(0.5+1j*0.3632);
V23=2/5*Vdc*(0.1909+1j*0.5877);
V24=2/5*Vdc*(-0.1909+1j*0.5877);
V25=2/5*Vdc*(-0.5+1j*0.3632);
V26=2/5*Vdc*(-0.6180+1j*0);
V27=2/5*Vdc*(-0.5-1j*0.3632);
V28=2/5*Vdc*(-0.1909-1j*0.5877);
V29=2/5*Vdc*(0.1909-1j*0.5877);
V30=2/5*Vdc*(0.5-1j*0.3632);
V31=0;
V32=0;
V=[V1 V2 V3 V4 V5 V6 V7 V8 V9 V10 V11 V12 V13 V14 V15 V16 V17 V18 V19 V20 V21 V22 V23 V24 V25 V26 V27 V28 V29 V30 V31 V32];
states=[1 1 0 0 1;
        1 1 0 0 0;
        1 1 1 0 0;
        0 1 1 0 0;
        0 1 1 1 0;
        0 0 1 1 0;
        0 0 1 1 1;
        0 0 0 1 1;
        1 0 0 1 1;
        1 0 0 0 1;
        1 0 0 0 0;
        1 1 1 0 1;
        0 1 0 0 0;
        1 1 1 1 0;
        0 0 1 0 0;
        0 1 1 1 1;
        0 0 0 1 0;
        1 0 1 1 1;
        0 0 0 0 1;
        1 1 0 1 1;
        0 1 0 0 1;
        1 1 0 1 0;
        1 0 1 0 0;
        0 1 1 0 1;
        0 1 0 1 0;
        1 0 1 1 0;
        0 0 1 0 1;
        0 1 0 1 1;
        1 0 0 1 0;
        1 0 1 0 1;
        0 0 0 0 0;
        1 1 1 1 1];       
H1=2/5*Vdc*(-0.6180+1j*0);
H2=2/5*Vdc*(0.1909-1j*0.5877);
H3=2/5*Vdc*(0.5+1j*0.3632);
H4=2/5*Vdc*(-0.5+1j*0.3632);
H5=2/5*Vdc*(-0.1909-1j*0.5877); 
H6=2/5*Vdc*(0.6180+1j*0); 
H7=2/5*Vdc*(-0.1909+1j*0.5877); 
H8=2/5*Vdc*(-0.5-1j*0.3632);
H9=2/5*Vdc*(0.5-1j*0.3632);
H10=2/5*Vdc*(0.1909+1j*0.5877);
H11=2/5*Vdc*(1+1j*0);
H12=2/5*Vdc*(-0.3090+1j*0.9510);
H13=2/5*Vdc*(-0.8090-1j*0.5877);
H14=2/5*Vdc*(0.8090-1j*0.5877);
H15=2/5*Vdc*(0.3090+1j*0.9510);
H16=2/5*Vdc*(-1+1j*0);
H17=2/5*Vdc*(0.3090-1j*0.9510);
H18=2/5*Vdc*(0.8090+1j*0.5877);
H19=2/5*Vdc*(-0.8090+1j*0.5877);
H20=2/5*Vdc*(-0.3090-1j*0.9510);
H21=2/5*Vdc*(-1.6180+1j*0);
H22=2/5*Vdc*(0.5-1j*1.5388);
H23=2/5*Vdc*(1.3090+1j*0.9510);
H24=2/5*Vdc*(-1.3090+1j*0.9510);
H25=2/5*Vdc*(-0.5-1j*1.5388);
H26=2/5*Vdc*(1.6180+1j*0);
H27=2/5*Vdc*(-0.5+1j*1.5388);
H28=2/5*Vdc*(-1.3090-1j*0.9510);
H29=2/5*Vdc*(1.3090-1j*0.9510);
H30=2/5*Vdc*(0.5+1j*1.5388); 
H31=0;
H32=0;
H=[H1 H2 H3 H4 H5 H6 H7 H8 H9 H10 H11 H12 H13 H14 H15 H16 H17 H18 H19 H20 H21 H22 H23 H24 H25 H26 H27 H28 H29 H30 H31 H32];
persistent x_opt 
if isempty(x_opt),x_opt=1;
end
is_ref=(Id1_ref+1j*Iq1_ref)*(cos(thetaR)+1j*sin(thetaR));
Iaplha_ref=real(is_ref);
Ibeta_ref=imag(is_ref);
Ix_ref=Id3_ref;
Iy_ref=Iq3_ref;
Ih=Id3+1j*Iq3;
g_opt=1e10;us=0;e0=0;     
for i=1:30
    V_o1 = V(i);
    H_o1 = H(i);
    Isp1 = i_meas+(Ts*(V_o1-(Rs*i_meas))/Ls)-((1j*Lamda_PM*Wr*Ts)*(cos(thetaR)+1j*sin(thetaR)))/Ls;
%     Isp01=Isp1-(V_o1*Ts/Ls);
    Ihp1 = (Ts/Lls)*(H_o1)+Ih*(1-(Rs*Ts/Lls));
    Iaplhap1=real(Isp1);
    Ibetap1=imag(Isp1);
    Ixp1=real(Ihp1);
    Iyp1=imag(Ihp1);
    g= (abs(Iaplha_ref - Iaplhap1))^2+ (abs(Ibeta_ref- Ibetap1))^2+(abs(Ix_ref - Ixp1))^2+(abs(Iy_ref - Iyp1))^2;
    if (g<g_opt)
        g_opt = g;
        x_opt = i;
        us=V_o1;
        e0=(Iaplha_ref+1j*Ibeta_ref)-Isp1;
    end
end
D=abs(dot(e0,Ts*us/Ls)/(dot((Ts*us/Ls),(Ts*us/Ls))));
if(D>1)
D=1;
end
DSa = D*states(x_opt,1);
DSb = D*states(x_opt,2);
DSc = D*states(x_opt,3);
DSd = D*states(x_opt,4);
DSe = D*states(x_opt,5);
d=D;
